simulink model "test7_blocks_named_port_orig"  (R2016b)
settings: Solver=VariableStepAuto  StartTime=0.0  StopTime=10.0  RelTol=1e-3
settings Model: Creator=gm  LastModifiedBy=gm

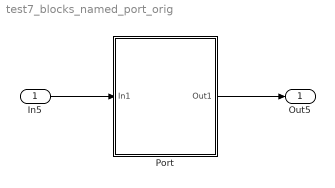
== system test7_blocks_named_port_orig ==
  In5 : Inport
  Port : Subsystem
  Out5 : Outport
  wires:
  In5/1 -> Port/1(In1)
  Port/1(Out1) -> Out5/1

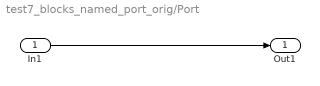
== system test7_blocks_named_port_orig/Port ==
  In1 : Inport
  Out1 : Outport
  wires:
  In1/1 -> Out1/1
